simulink subsystem "rss_FaltEnFlgConfSens"  (R2023a)
settings: Solver=VariableStepAuto  StartTime=0.0  StopTime=10.0  RelTol=1e-3
undefined symbols (not defined in the file): Cdbl_numFaltDiaNum, ENM_SYS_STATUS, Gbol_flgFaltManEnFlg_C, Gu16_uComDiaDisblHiLvlConfTrs_C, Gu16_uComDiaDisblHiLvlRcvyTrs_C, Gu16_uComDiaDisblLoLvlConfTrs_C, Gu16_uComDiaDisblLoLvlRcvyTrs_C, Gu8_ctComDiaDisblHiLvlConfCnt_C, Gu8_ctComDiaDisblHiLvlRcvyCnt_C, Gu8_ctComDiaDisblLoLvlConfCnt_C, Gu8_ctComDiaDisblLoLvlRcvyCnt_C
libraries: simulink x3, lib_hysteresis_debounce x2
settings Model: Creator=xiaoqiang.yuan  LastModifiedBy=xiaoqiang.yuan

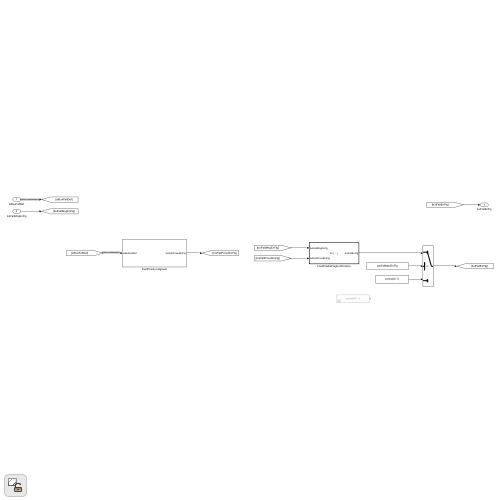
[thumbnail: Simulink's stored preview of the top-level diagram]
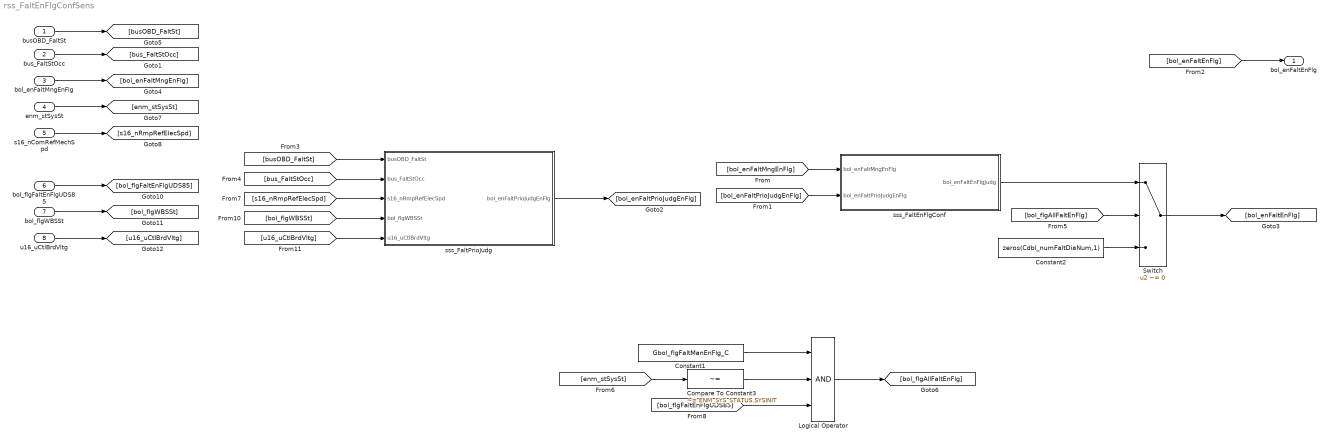
== system rss_FaltEnFlgConfSens ==
  busOBD_FaltSt : Inport
  bus_FaltStOcc : Inport  Port=2
  bol_enFaltMngEnFlg : Inport  Port=3
  enm_stSysSt : Inport  Port=4  OutDataTypeStr=Enum: ENM_SYS_STATUS
  s16_nComRefMechSpd : Inport  Port=5  OutDataTypeStr=dt_Standardize_s16p15b0
  bol_flgFaltEnFlgUDS85 : Inport  Port=6  OutDataTypeStr=boolean
  bol_flgWBSSt : Inport  Port=7  OutDataTypeStr=boolean
  u16_uCtlBrdVltg : Inport  Port=8  OutDataTypeStr=dt_Standardize_u16p15b0
  Compare To Constant3 : simulink/Logic and Bit Operations/Compare To Constant  relop=~=  const=ENM_SYS_STATUS.SYSINIT  OutDataTypeStr=boolean
  Constant1 : Constant  Value=Gbol_flgFaltManEnFlg_C
  Constant2 : Constant  Value=zeros(Cdbl_numFaltDiaNum,1)  OutDataTypeStr=boolean
  Logical Operator : Logic  Inputs=3  AllPortsSameDT=off  OutDataTypeStr=boolean
  Switch : Switch  Criteria=u2 ~= 0  SaturateOnIntegerOverflow=off  InputSameDT=off
  sss_FaltEnFlgConf : Subsystem  TreatAsAtomicUnit=on
      settings: RTWSystemCode=Nonreusable function
  sss_FaltPrioJudg : Subsystem
  bol_enFaltEnFlg : Outport
  wires:
  busOBD_FaltSt/1 -> [busOBD_FaltSt]
  [busOBD_FaltSt] -> sss_FaltPrioJudg/1(busOBD_FaltSt)
  sss_FaltPrioJudg/1(bol_enFaltPrioJudgEnFlg) -> [bol_enFaltPrioJudgEnFlg]
  [bol_enFaltMngEnFlg] -> sss_FaltEnFlgConf/1(bol_enFaltMngEnFlg)
  [bol_enFaltPrioJudgEnFlg] -> sss_FaltEnFlgConf/2(bol_enFaltPrioJudgEnFlg)
  [bol_enFaltEnFlg] -> bol_enFaltEnFlg/1
  bol_enFaltMngEnFlg/1 -> [bol_enFaltMngEnFlg]
  Constant2/1 -> Switch/3
  Switch/1 -> [bol_enFaltEnFlg]
  sss_FaltEnFlgConf/1(bol_enFaltEnFlgJudg) -> Switch/1
  bus_FaltStOcc/1 -> [bus_FaltStOcc]
  [bus_FaltStOcc] -> sss_FaltPrioJudg/2(bus_FaltStOcc)
  [bol_flgAllFaltEnFlg] -> Switch/2
  Constant1/1 -> Logical Operator/1
  enm_stSysSt/1 -> [enm_stSysSt]
  [enm_stSysSt] -> Compare To Constant3/1
  Compare To Constant3/1 -> Logical Operator/2
  Logical Operator/1 -> [bol_flgAllFaltEnFlg]
  s16_nComRefMechSpd/1 -> [s16_nRmpRefElecSpd]
  [s16_nRmpRefElecSpd] -> sss_FaltPrioJudg/3(s16_nRmpRefElecSpd)
  bol_flgFaltEnFlgUDS85/1 -> [bol_flgFaltEnFlgUDS85]
  bol_flgWBSSt/1 -> [bol_flgWBSSt]
  [bol_flgFaltEnFlgUDS85] -> Logical Operator/3
  u16_uCtlBrdVltg/1 -> [u16_uCtlBrdVltg]
  [bol_flgWBSSt] -> sss_FaltPrioJudg/4(bol_flgWBSSt)
  [u16_uCtlBrdVltg] -> sss_FaltPrioJudg/5(u16_uCtlBrdVltg)

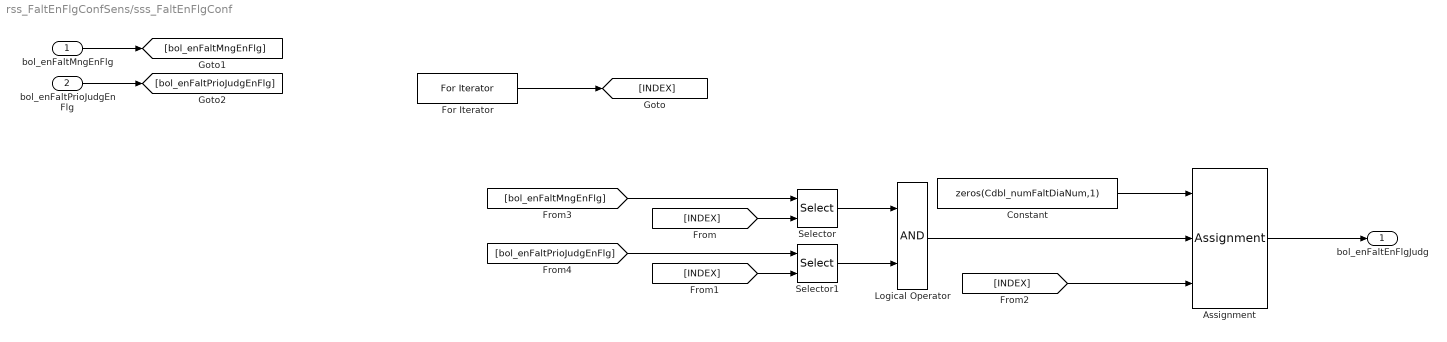
== system rss_FaltEnFlgConfSens/sss_FaltEnFlgConf ==
  bol_enFaltMngEnFlg : Inport
  bol_enFaltPrioJudgEnFlg : Inport  Port=2
  Assignment : Assignment  DiagnosticForDimensions=Warning  IndexOptions=Index vector (port)  Indices=1  OutputSizes=1
  Constant : Constant  Value=zeros(Cdbl_numFaltDiaNum,1)  OutDataTypeStr=boolean
  For Iterator : ForIterator  IterationLimit=Cdbl_numFaltDiaNum  IterationVariableDataType=uint8
  Logical Operator : Logic  AllPortsSameDT=off  OutDataTypeStr=boolean
  Selector : Selector  InputPortWidth=Cdbl_numFaltDiaNum  IndexOptions=Index vector (port)  Indices=[1 3]  OutputSizes=1
  Selector1 : Selector  InputPortWidth=Cdbl_numFaltDiaNum  IndexOptions=Index vector (port)  Indices=[1 3]  OutputSizes=1
  bol_enFaltEnFlgJudg : Outport
  wires:
  Assignment/1 -> bol_enFaltEnFlgJudg/1
  [bol_enFaltPrioJudgEnFlg] -> Selector1/1
  bol_enFaltPrioJudgEnFlg/1 -> [bol_enFaltPrioJudgEnFlg]
  bol_enFaltMngEnFlg/1 -> [bol_enFaltMngEnFlg]
  Selector/1 -> Logical Operator/1
  [bol_enFaltMngEnFlg] -> Selector/1
  For Iterator/1 -> [INDEX]
  [INDEX] -> Selector/2
  [INDEX] -> Selector1/2
  Selector1/1 -> Logical Operator/2
  Logical Operator/1 -> Assignment/2
  Constant/1 -> Assignment/1
  [INDEX] -> Assignment/3

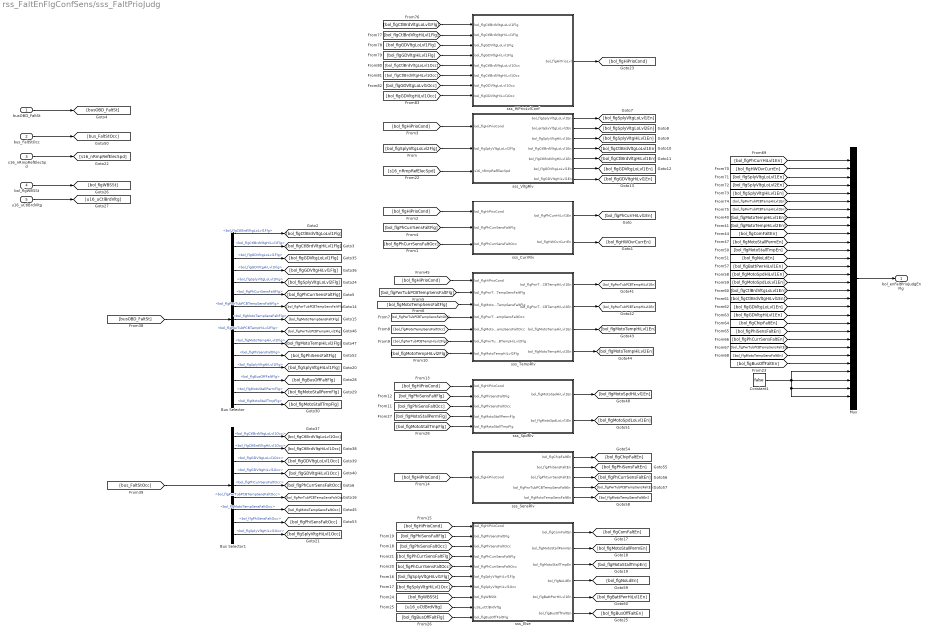
== system rss_FaltEnFlgConfSens/sss_FaltPrioJudg ==
  busOBD_FaltSt : Inport
  bus_FaltStOcc : Inport  Port=2
  s16_nRmpRefElecSpd : Inport  Port=3
  bol_flgWBSSt : Inport  Port=4
  u16_uCtlBrdVltg : Inport  Port=5
  Bus Selector : BusSelector  OutputSignals=bol_flgCtlBrdVltgLoLvl1Flg,bol_flgCtlBrdVltgHiLvl1Flg,bol_flgGDVltgLoLvl1Flg,bol_flgGDVltgHiLvl1Flg,bol_flgSplyVltgLoLvl2Flg,bol_flgPhCurrSensFaltFlg,bol_flgPwrTubPCBTempSensFaltFlg,bol_flgMotoTempSensFaltFlg,bol_flgPwrTubPCBTempHiLvl2Flg,bol_flgMotoTempHiLvl2Flg,bol_flgPhiSensFaltFlg,bol_flgSplyVltgHiLvl1Flg,bol_flgBusOffFaltFlg,bol_flgMotoStallPermFlg,bol_flgMotoStallTmpFlg
  Bus Selector1 : BusSelector  OutputSignals=bol_flgCtlBrdVltgLoLvl1Occ,bol_flgCtlBrdVltgHiLvl1Occ,bol_flgGDVltgLoLvl1Occ,bol_flgGDVltgHiLvl1Occ,bol_flgPhCurrSensFaltOcc,bol_flgPwrTubPCBTempSensFaltOcc,bol_flgMotoTempSensFaltOcc,bol_flgPhiSensFaltOcc,bol_flgSplyVltgHiLvl1Occ
  Constant1 : Constant  Value=false  OutDataTypeStr=boolean
  Mux : Mux  Inputs=30
  sss_CurrRlv : Subsystem
  sss_Else : Subsystem
  sss_HiPrioLvlConf : Subsystem
  sss_SensRlv : Subsystem
  sss_SpdRlv : Subsystem
  sss_TempRlv : Subsystem
  sss_VltgRlv : Subsystem
  bol_enFaltPrioJudgEnFlg : Outport
  wires:
  [bol_flgMotoStallTmpFlg] -> sss_SpdRlv/5(bol_flgMotoStallTmpFlg)
  [bol_flgMotoStallPermFlg] -> sss_SpdRlv/4(bol_flgMotoStallPermFlg)
  Bus Selector/15 -> [bol_flgMotoStallTmpFlg]  "<bol_flgMotoStallTmpFlg>"
  Bus Selector/14 -> [bol_flgMotoStallPermFlg]  "<bol_flgMotoStallPermFlg>"
  [bol_flgBusOffFaltEn] -> Mux/26
  sss_Else/6(bol_flgBusOffFaltEn) -> [bol_flgBusOffFaltEn]
  [bol_flgBusOffFaltFlg] -> sss_Else/10(bol_flgBusOffFaltFlg)
  Bus Selector/13 -> [bol_flgBusOffFaltFlg]  "<bol_flgBusOffFaltFlg>"
  [u16_uCtlBrdVltg] -> sss_Else/9(u16_uCtlBrdVltg)
  [bol_flgWBSSt] -> sss_Else/8(bol_flgWBSSt)
  u16_uCtlBrdVltg/1 -> [u16_uCtlBrdVltg]
  bol_flgWBSSt/1 -> [bol_flgWBSSt]
  [s16_nRmpRefElecSpd] -> sss_VltgRlv/3(s16_nRmpRefElecSpd)
  s16_nRmpRefElecSpd/1 -> [s16_nRmpRefElecSpd]
  [bol_flgSplyVltgHiLvl1Occ] -> sss_Else/7(bol_flgSplyVltgHiLvl1Occ)
  [bol_flgSplyVltgHiLvl1Flg] -> sss_Else/6(bol_flgSplyVltgHiLvl1Flg)
  [bol_flgPhCurrSensFaltOcc] -> sss_Else/5(bol_flgPhCurrSensFaltOcc)
  [bol_flgPhCurrSensFaltFlg] -> sss_Else/4(bol_flgPhCurrSensFaltFlg)
  [bol_flgPhiSensFaltOcc] -> sss_Else/3(bol_flgPhiSensFaltOcc)
  [bol_flgPhiSensFaltFlg] -> sss_Else/2(bol_flgPhiSensFaltFlg)
  Bus Selector1/9 -> [bol_flgSplyVltgHiLvl1Occ]  "<bol_flgSplyVltgHiLvl1Occ>"
  Bus Selector/12 -> [bol_flgSplyVltgHiLvl1Flg]  "<bol_flgSplyVltgHiLvl1Flg>"
  [bol_flgHiPrioCond] -> sss_Else/1(bol_flgHiPrioCond)
  sss_Else/5(bol_flgBattPwrHiLvl1En) -> [bol_flgBattPwrHiLvl1En]
  sss_Else/4(bol_flgNoLdEn) -> [bol_flgNoLdEn]
  sss_Else/3(bol_flgMotoStallTmpEn) -> [bol_flgMotoStallTmpEn]
  sss_Else/2(bol_flgMotoStallPermEn) -> [bol_flgMotoStallPermEn]
  sss_Else/1(bol_flgComFaltEn) -> [bol_flgComFaltEn]
  sss_SensRlv/5(bol_flgMotoTempSensFaltEn) -> [bol_flgMotoTempSensFaltEn]
  sss_SensRlv/4(bol_flgPwrTubPCBTempSensFaltEn) -> [bol_flgPwrTubPCBTempSensFaltEn]
  sss_SensRlv/3(bol_flgPhCurrSensFaltEn) -> [bol_flgPhCurrSensFaltEn]
  sss_SensRlv/2(bol_flgPhiSensFaltEn) -> [bol_flgPhiSensFaltEn]
  sss_SensRlv/1(bol_flgChipFaltEn) -> [bol_flgChipFaltEn]
  [bol_flgHiPrioCond] -> sss_SensRlv/1(bol_flgHiPrioCond)
  [bol_flgPhiSensFaltFlg] -> sss_SpdRlv/2(bol_flgPhiSensFaltFlg)
  [bol_flgPhiSensFaltOcc] -> sss_SpdRlv/3(bol_flgPhiSensFaltOcc)
  [bol_flgHiPrioCond] -> sss_SpdRlv/1(bol_flgHiPrioCond)
  Bus Selector1/8 -> [bol_flgPhiSensFaltOcc]  "<bol_flgPhiSensFaltOcc>"
  Bus Selector/11 -> [bol_flgPhiSensFaltFlg]  "<bol_flgPhiSensFaltFlg>"
  sss_SpdRlv/2(bol_flgMotoSpdLoLvl1En) -> [bol_flgMotoSpdLoLvl1En]
  sss_SpdRlv/1(bol_flgMotoSpdHiLvl1En) -> [bol_flgMotoSpdHiLvl1En]
  Bus Selector/10 -> [bol_flgMotoTempHiLvl2Flg]  "<bol_flgMotoTempHiLvl2Flg>"
  Bus Selector/9 -> [bol_flgPwrTubPCBTempHiLvl2Flg]  "<bol_flgPwrTubPCBTempHiLvl2Flg>"
  sss_TempRlv/1(bol_flgPwrTubPCBTempHiLvl1En) -> [bol_flgPwrTubPCBTempHiLvl1En]
  sss_TempRlv/2(bol_flgPwrTubPCBTempHiLvl2En) -> [bol_flgPwrTubPCBTempHiLvl2En]
  sss_TempRlv/3(bol_flgMotoTempHiLvl1En) -> [bol_flgMotoTempHiLvl1En]
  sss_TempRlv/4(bol_flgMotoTempHiLvl2En) -> [bol_flgMotoTempHiLvl2En]
  [bol_flgMotoTempHiLvl2Flg] -> sss_TempRlv/7(bol_flgMotoTempHiLvl2Flg)
  [bol_flgPwrTubPCBTempHiLvl2Flg] -> sss_TempRlv/6(bol_flgPwrTubPCBTempHiLvl2Flg)
  [bol_flgMotoTempSensFaltOcc] -> sss_TempRlv/5(bol_flgMotoTempSensFaltOcc)
  [bol_flgPwrTubPCBTempSensFaltOcc] -> sss_TempRlv/4(bol_flgPwrTubPCBTempSensFaltOcc)
  [bol_flgMotoTempSensFaltFlg] -> sss_TempRlv/3(bol_flgMotoTempSensFaltFlg)
  [bol_flgPwrTubPCBTempSensFaltFlg] -> sss_TempRlv/2(bol_flgPwrTubPCBTempSensFaltFlg)
  Bus Selector1/7 -> [bol_flgMotoTempSensFaltOcc]  "<bol_flgMotoTempSensFaltOcc>"
  Bus Selector1/6 -> [bol_flgPwrTubPCBTempSensFaltOcc]  "<bol_flgPwrTubPCBTempSensFaltOcc>"
  Bus Selector/8 -> [bol_flgMotoTempSensFaltFlg]  "<bol_flgMotoTempSensFaltFlg>"
  Bus Selector/7 -> [bol_flgPwrTubPCBTempSensFaltFlg]  "<bol_flgPwrTubPCBTempSensFaltFlg>"
  [bol_flgHiPrioCond] -> sss_CurrRlv/1(bol_flgHiPrioCond)
  [bol_flgPhCurrSensFaltOcc] -> sss_CurrRlv/3(bol_flgPhCurrSensFaltOcc)
  [bol_flgPhCurrSensFaltFlg] -> sss_CurrRlv/2(bol_flgPhCurrSensFaltFlg)
  Bus Selector1/5 -> [bol_flgPhCurrSensFaltOcc]  "<bol_flgPhCurrSensFaltOcc>"
  Bus Selector/6 -> [bol_flgPhCurrSensFaltFlg]  "<bol_flgPhCurrSensFaltFlg>"
  [bol_flgSplyVltgLoLvl2Flg] -> sss_VltgRlv/2(bol_flgSplyVltgLoLvl2Flg)
  Bus Selector/5 -> [bol_flgSplyVltgLoLvl2Flg]  "<bol_flgSplyVltgLoLvl2Flg>"
  [bol_flgHiPrioCond] -> sss_VltgRlv/1(bol_flgHiPrioCond)
  sss_VltgRlv/7(bol_flgGDVltgHiLvl1En) -> [bol_flgGDVltgHiLvl1En]
  sss_VltgRlv/6(bol_flgGDVltgLoLvl1En) -> [bol_flgGDVltgLoLvl1En]
  sss_VltgRlv/5(bol_flgCtlBrdVltgHiLvl1En) -> [bol_flgCtlBrdVltgHiLvl1En]
  sss_VltgRlv/4(bol_flgCtlBrdVltgLoLvl1En) -> [bol_flgCtlBrdVltgLoLvl1En]
  sss_VltgRlv/3(bol_flgSplyVltgHiLvl1En) -> [bol_flgSplyVltgHiLvl1En]
  sss_VltgRlv/2(bol_enSplyVltgLoLvl2En) -> [bol_flgSplyVltgLoLvl2En]
  sss_VltgRlv/1(bol_flgSplyVltgLoLvl1En) -> [bol_flgSplyVltgLoLvl1En]
  Mux/1 -> bol_enFaltPrioJudgEnFlg/1
  [bol_flgGDVltgHiLvl1Occ] -> sss_HiPrioLvlConf/8(bol_flgGDVltgHiLvl1Occ)
  [bol_flgGDVltgLoLvl1Occ] -> sss_HiPrioLvlConf/7(bol_flgGDVltgLoLvl1Occ)
  [bol_flgCtlBrdVltgHiLvl1Occ] -> sss_HiPrioLvlConf/6(bol_flgCtlBrdVltgHiLvl1Occ)
  [bol_flgCtlBrdVltgLoLvl1Occ] -> sss_HiPrioLvlConf/5(bol_flgCtlBrdVltgLoLvl1Occ)
  [bol_flgGDVltgHiLvl1Flg] -> sss_HiPrioLvlConf/4(bol_flgGDVltgHiLvl1Flg)
  [bol_flgGDVltgLoLvl1Flg] -> sss_HiPrioLvlConf/3(bol_flgGDVltgLoLvl1Flg)
  [bol_flgCtlBrdVltgHiLvl1Flg] -> sss_HiPrioLvlConf/2(bol_flgCtlBrdVltgHiLvl1Flg)
  [bol_flgCtlBrdVltgLoLvl1Flg] -> sss_HiPrioLvlConf/1(bol_flgCtlBrdVltgLoLvl1Flg)
  Bus Selector1/4 -> [bol_flgGDVltgHiLvl1Occ]  "<bol_flgGDVltgHiLvl1Occ>"
  Bus Selector1/3 -> [bol_flgGDVltgLoLvl1Occ]  "<bol_flgGDVltgLoLvl1Occ>"
  Bus Selector1/2 -> [bol_flgCtlBrdVltgHiLvl1Occ]  "<bol_flgCtlBrdVltgHiLvl1Occ>"
  Bus Selector1/1 -> [bol_flgCtlBrdVltgLoLvl1Occ]  "<bol_flgCtlBrdVltgLoLvl1Occ>"
  [bol_flgGDVltgHiLvl1En] -> Mux/20
  [bol_flgMotoStallPermEn] -> Mux/11
  [bol_flgPhCurrSensFaltEn] -> Mux/23
  [bol_flgCtlBrdVltgHiLvl1En] -> Mux/18
  [bol_flgMotoStallTmpEn] -> Mux/12
  [bol_flgMotoSpdLoLvl1En] -> Mux/16
  [bol_flgCtlBrdVltgLoLvl1En] -> Mux/17
  [bol_flgBattPwrHiLvl1En] -> Mux/14
  [bol_flgNoLdEn] -> Mux/13
  [bol_flgPhCurrHiLvl1En] -> Mux/1
  [bol_flgPhiSensFaltEn] -> Mux/22
  [bol_flgMotoTempHiLvl1En] -> Mux/8
  [bol_flgMotoTempHiLvl2En] -> Mux/9
  [bol_flgChipFaltEn] -> Mux/21
  [bol_flgHWOvrCurrEn] -> Mux/2
  [bol_flgPwrTubPCBTempHiLvl1En] -> Mux/6
  [bol_flgComFaltEn] -> Mux/10
  [bol_flgPwrTubPCBTempHiLvl2En] -> Mux/7
  [bol_flgMotoSpdHiLvl1En] -> Mux/15
  [bol_flgSplyVltgHiLvl1En] -> Mux/5
  [bol_flgPwrTubPCBTempSensFaltEn] -> Mux/24
  [bol_flgGDVltgLoLvl1En] -> Mux/19
  [bol_flgSplyVltgLoLvl2En] -> Mux/4
  [bol_flgMotoTempSensFaltEn] -> Mux/25
  [bol_flgSplyVltgLoLvl1En] -> Mux/3
  Constant1/1 -> Mux/30, Mux/29, Mux/28, Mux/27
  [bus_FaltStOcc] -> Bus Selector1/1
  bus_FaltStOcc/1 -> [bus_FaltStOcc]
  sss_HiPrioLvlConf/1(bol_flgHiPrioLvl) -> [bol_flgHiPrioCond]
  [bol_flgHiPrioCond] -> sss_TempRlv/1(bol_flgHiPrioCond)
  sss_CurrRlv/2(bol_flgHWOvrCurrEn) -> [bol_flgHWOvrCurrEn]
  sss_CurrRlv/1(bol_flgPhCurrHiLvl1En) -> [bol_flgPhCurrHiLvl1En]
  Bus Selector/4 -> [bol_flgGDVltgHiLvl1Flg]  "<bol_flgGDVltgHiLvl1Flg>"
  Bus Selector/3 -> [bol_flgGDVltgLoLvl1Flg]  "<bol_flgGDVltgLoLvl1Flg>"
  busOBD_FaltSt/1 -> [busOBD_FaltSt]
  Bus Selector/2 -> [bol_flgCtlBrdVltgHiLvl1Flg]  "<bol_flgCtlBrdVltgHiLvl1Flg>"
  Bus Selector/1 -> [bol_flgCtlBrdVltgLoLvl1Flg]  "<bol_flgCtlBrdVltgLoLvl1Flg>"
  [busOBD_FaltSt] -> Bus Selector/1

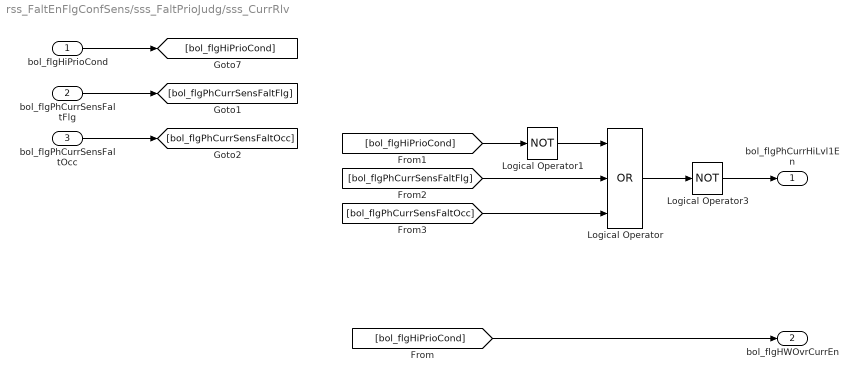
== system rss_FaltEnFlgConfSens/sss_FaltPrioJudg/sss_CurrRlv ==
  bol_flgHiPrioCond : Inport
  bol_flgPhCurrSensFaltFlg : Inport  Port=2
  bol_flgPhCurrSensFaltOcc : Inport  Port=3
  Logical Operator : Logic  Operator=OR  Inputs=3  AllPortsSameDT=off  OutDataTypeStr=boolean
  Logical Operator1 : Logic  Operator=NOT  AllPortsSameDT=off  OutDataTypeStr=boolean
  Logical Operator3 : Logic  Operator=NOT  AllPortsSameDT=off  OutDataTypeStr=boolean
  bol_flgPhCurrHiLvl1En : Outport
  bol_flgHWOvrCurrEn : Outport  Port=2
  wires:
  [bol_flgPhCurrSensFaltOcc] -> Logical Operator/3
  [bol_flgHiPrioCond] -> Logical Operator1/1
  Logical Operator3/1 -> bol_flgPhCurrHiLvl1En/1
  bol_flgPhCurrSensFaltOcc/1 -> [bol_flgPhCurrSensFaltOcc]
  bol_flgPhCurrSensFaltFlg/1 -> [bol_flgPhCurrSensFaltFlg]
  bol_flgHiPrioCond/1 -> [bol_flgHiPrioCond]
  Logical Operator/1 -> Logical Operator3/1
  [bol_flgHiPrioCond] -> bol_flgHWOvrCurrEn/1
  [bol_flgPhCurrSensFaltFlg] -> Logical Operator/2
  Logical Operator1/1 -> Logical Operator/1

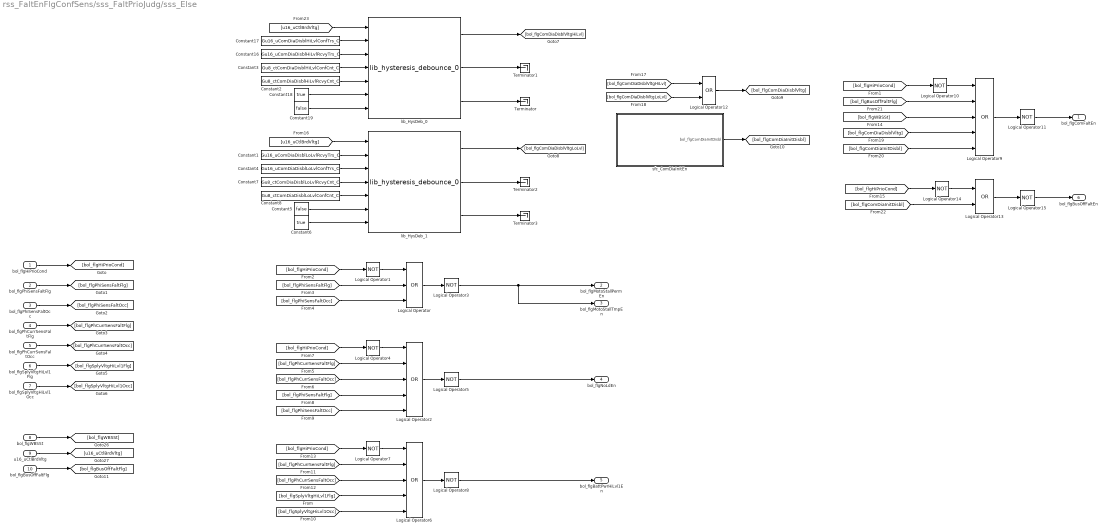
== system rss_FaltEnFlgConfSens/sss_FaltPrioJudg/sss_Else ==
  bol_flgHiPrioCond : Inport
  bol_flgPhiSensFaltFlg : Inport  Port=2
  bol_flgPhiSensFaltOcc : Inport  Port=3
  bol_flgPhCurrSensFaltFlg : Inport  Port=4
  bol_flgPhCurrSensFaltOcc : Inport  Port=5
  bol_flgSplyVltgHiLvl1Flg : Inport  Port=6
  bol_flgSplyVltgHiLvl1Occ : Inport  Port=7
  bol_flgWBSSt : Inport  Port=8
  u16_uCtlBrdVltg : Inport  Port=9
  bol_flgBusOffFaltFlg : Inport  Port=10
  Constant1 : Constant  Value=Gu16_uComDiaDisblLoLvlRcvyTrs_C
  Constant16 : Constant  Value=Gu16_uComDiaDisblHiLvlRcvyTrs_C
  Constant17 : Constant  Value=Gu16_uComDiaDisblHiLvlConfTrs_C
  Constant18 : Constant  Value=true  OutDataTypeStr=boolean
  Constant19 : Constant  Value=false  OutDataTypeStr=boolean
  Constant2 : Constant  Value=Gu8_ctComDiaDisblHiLvlRcvyCnt_C
  Constant3 : Constant  Value=Gu8_ctComDiaDisblHiLvlConfCnt_C
  Constant4 : Constant  Value=Gu16_uComDiaDisblLoLvlConfTrs_C
  Constant5 : Constant  Value=false  OutDataTypeStr=boolean
  Constant6 : Constant  Value=true  OutDataTypeStr=boolean
  Constant7 : Constant  Value=Gu8_ctComDiaDisblLoLvlRcvyCnt_C
  Constant8 : Constant  Value=Gu8_ctComDiaDisblLoLvlConfCnt_C
  Logical Operator : Logic  Operator=OR  Inputs=3  AllPortsSameDT=off  OutDataTypeStr=boolean
  Logical Operator{1,3..5,7..8,10..11,14..15} (10 alike) : Logic  Operator=NOT  AllPortsSameDT=off  OutDataTypeStr=boolean
  Logical Operator12 : Logic  Operator=OR  AllPortsSameDT=off  OutDataTypeStr=boolean
  Logical Operator13 : Logic  Operator=OR  AllPortsSameDT=off  OutDataTypeStr=boolean
  Logical Operator2 : Logic  Operator=OR  Inputs=5  AllPortsSameDT=off  OutDataTypeStr=boolean
  Logical Operator6 : Logic  Operator=OR  Inputs=5  AllPortsSameDT=off  OutDataTypeStr=boolean
  Logical Operator9 : Logic  Operator=OR  Inputs=5  AllPortsSameDT=off  OutDataTypeStr=boolean
  Terminator{,1..3} (4 alike) : Terminator
  lib_HysDeb_0 : lib_hysteresis_debounce/lib_hysteresis_debounce_0  lb_parInitOutp=0
  lib_HysDeb_1 : lib_hysteresis_debounce/lib_hysteresis_debounce_0  lb_parInitOutp=0
  sfc_ComDiaInitEn : Stateflow chart  TreatAsAtomicUnit=on
  bol_flgComFaltEn : Outport
  bol_flgMotoStallPermEn : Outport  Port=2
  bol_flgMotoStallTmpEn : Outport  Port=3
  bol_flgNoLdEn : Outport  Port=4
  bol_flgBattPwrHiLvl1En : Outport  Port=5
  bol_flgBusOffFaltEn : Outport  Port=6
  wires:
  Logical Operator15/1 -> bol_flgBusOffFaltEn/1
  Logical Operator14/1 -> Logical Operator13/1
  [bol_flgHiPrioCond] -> Logical Operator14/1
  Logical Operator13/1 -> Logical Operator15/1
  [bol_flgComDiaInitDisbl] -> Logical Operator13/2
  [bol_flgBusOffFaltFlg] -> Logical Operator9/2
  bol_flgBusOffFaltFlg/1 -> [bol_flgBusOffFaltFlg]
  sfc_ComDiaInitEn/1(bol_flgComDiaInitDisbl) -> [bol_flgComDiaInitDisbl]
  [bol_flgComDiaInitDisbl] -> Logical Operator9/5
  Logical Operator11/1 -> bol_flgComFaltEn/1
  [bol_flgComDiaDisblVltg] -> Logical Operator9/4
  Logical Operator12/1 -> [bol_flgComDiaDisblVltg]
  [bol_flgComDiaDisblVltgHiLvl] -> Logical Operator12/1
  [bol_flgComDiaDisblVltgLoLvl] -> Logical Operator12/2
  lib_HysDeb_1/2 -> Terminator2/1
  Constant6/1 -> lib_HysDeb_1/7
  lib_HysDeb_1/1 -> [bol_flgComDiaDisblVltgLoLvl]
  Constant7/1 -> lib_HysDeb_1/4
  Constant1/1 -> lib_HysDeb_1/2
  Constant5/1 -> lib_HysDeb_1/6
  Constant4/1 -> lib_HysDeb_1/3
  [u16_uCtlBrdVltg] -> lib_HysDeb_1/1
  Constant8/1 -> lib_HysDeb_1/5
  lib_HysDeb_1/3 -> Terminator3/1
  [u16_uCtlBrdVltg] -> lib_HysDeb_0/1
  lib_HysDeb_0/1 -> [bol_flgComDiaDisblVltgHiLvl]
  Constant19/1 -> lib_HysDeb_0/7
  Constant18/1 -> lib_HysDeb_0/6
  Constant16/1 -> lib_HysDeb_0/3
  lib_HysDeb_0/2 -> Terminator1/1
  lib_HysDeb_0/3 -> Terminator/1
  Constant3/1 -> lib_HysDeb_0/4
  Constant2/1 -> lib_HysDeb_0/5
  Constant17/1 -> lib_HysDeb_0/2
  Logical Operator10/1 -> Logical Operator9/1
  [bol_flgHiPrioCond] -> Logical Operator10/1
  Logical Operator9/1 -> Logical Operator11/1
  [bol_flgWBSSt] -> Logical Operator9/3
  bol_flgWBSSt/1 -> [bol_flgWBSSt]
  u16_uCtlBrdVltg/1 -> [u16_uCtlBrdVltg]
  [bol_flgSplyVltgHiLvl1Flg] -> Logical Operator6/4
  Logical Operator8/1 -> bol_flgBattPwrHiLvl1En/1
  [bol_flgHiPrioCond] -> Logical Operator7/1
  Logical Operator6/1 -> Logical Operator8/1
  [bol_flgPhCurrSensFaltFlg] -> Logical Operator6/2
  [bol_flgPhCurrSensFaltOcc] -> Logical Operator6/3
  Logical Operator7/1 -> Logical Operator6/1
  [bol_flgSplyVltgHiLvl1Occ] -> Logical Operator6/5
  bol_flgSplyVltgHiLvl1Occ/1 -> [bol_flgSplyVltgHiLvl1Occ]
  bol_flgSplyVltgHiLvl1Flg/1 -> [bol_flgSplyVltgHiLvl1Flg]
  [bol_flgPhiSensFaltOcc] -> Logical Operator2/5
  [bol_flgPhiSensFaltFlg] -> Logical Operator2/4
  [bol_flgHiPrioCond] -> Logical Operator4/1
  Logical Operator2/1 -> Logical Operator5/1
  Logical Operator5/1 -> bol_flgNoLdEn/1
  [bol_flgPhCurrSensFaltOcc] -> Logical Operator2/3
  [bol_flgPhCurrSensFaltFlg] -> Logical Operator2/2
  Logical Operator4/1 -> Logical Operator2/1
  bol_flgPhCurrSensFaltOcc/1 -> [bol_flgPhCurrSensFaltOcc]
  bol_flgPhCurrSensFaltFlg/1 -> [bol_flgPhCurrSensFaltFlg]
  Logical Operator3/1 -> bol_flgMotoStallPermEn/1, bol_flgMotoStallTmpEn/1
  [bol_flgPhiSensFaltOcc] -> Logical Operator/3
  [bol_flgPhiSensFaltFlg] -> Logical Operator/2
  bol_flgPhiSensFaltOcc/1 -> [bol_flgPhiSensFaltOcc]
  bol_flgPhiSensFaltFlg/1 -> [bol_flgPhiSensFaltFlg]
  Logical Operator/1 -> Logical Operator3/1
  [bol_flgHiPrioCond] -> Logical Operator1/1
  Logical Operator1/1 -> Logical Operator/1
  bol_flgHiPrioCond/1 -> [bol_flgHiPrioCond]

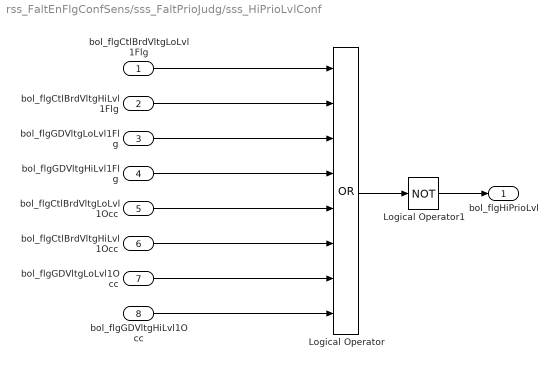
== system rss_FaltEnFlgConfSens/sss_FaltPrioJudg/sss_HiPrioLvlConf ==
  bol_flgCtlBrdVltgLoLvl1Flg : Inport
  bol_flgCtlBrdVltgHiLvl1Flg : Inport  Port=2
  bol_flgGDVltgLoLvl1Flg : Inport  Port=3
  bol_flgGDVltgHiLvl1Flg : Inport  Port=4
  bol_flgCtlBrdVltgLoLvl1Occ : Inport  Port=5
  bol_flgCtlBrdVltgHiLvl1Occ : Inport  Port=6
  bol_flgGDVltgLoLvl1Occ : Inport  Port=7
  bol_flgGDVltgHiLvl1Occ : Inport  Port=8
  Logical Operator : Logic  Operator=OR  Inputs=8  AllPortsSameDT=off  OutDataTypeStr=boolean
  Logical Operator1 : Logic  Operator=NOT  AllPortsSameDT=off  OutDataTypeStr=boolean
  bol_flgHiPrioLvl : Outport
  wires:
  Logical Operator1/1 -> bol_flgHiPrioLvl/1
  Logical Operator/1 -> Logical Operator1/1
  bol_flgGDVltgHiLvl1Occ/1 -> Logical Operator/8
  bol_flgGDVltgLoLvl1Occ/1 -> Logical Operator/7
  bol_flgCtlBrdVltgHiLvl1Occ/1 -> Logical Operator/6
  bol_flgCtlBrdVltgLoLvl1Occ/1 -> Logical Operator/5
  bol_flgGDVltgHiLvl1Flg/1 -> Logical Operator/4
  bol_flgGDVltgLoLvl1Flg/1 -> Logical Operator/3
  bol_flgCtlBrdVltgHiLvl1Flg/1 -> Logical Operator/2
  bol_flgCtlBrdVltgLoLvl1Flg/1 -> Logical Operator/1

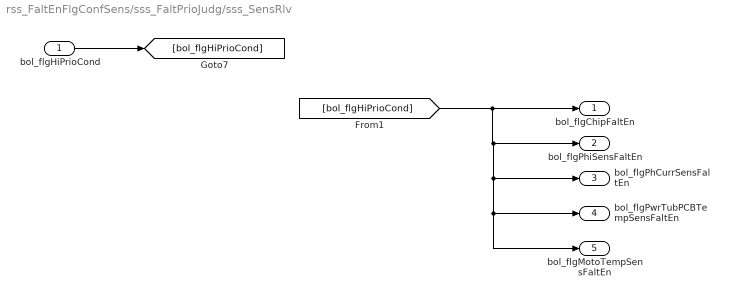
== system rss_FaltEnFlgConfSens/sss_FaltPrioJudg/sss_SensRlv ==
  bol_flgHiPrioCond : Inport
  bol_flgChipFaltEn : Outport
  bol_flgPhiSensFaltEn : Outport  Port=2
  bol_flgPhCurrSensFaltEn : Outport  Port=3
  bol_flgPwrTubPCBTempSensFaltEn : Outport  Port=4
  bol_flgMotoTempSensFaltEn : Outport  Port=5
  wires:
  [bol_flgHiPrioCond] -> bol_flgChipFaltEn/1, bol_flgPhiSensFaltEn/1, bol_flgPhCurrSensFaltEn/1, bol_flgMotoTempSensFaltEn/1, bol_flgPwrTubPCBTempSensFaltEn/1
  bol_flgHiPrioCond/1 -> [bol_flgHiPrioCond]

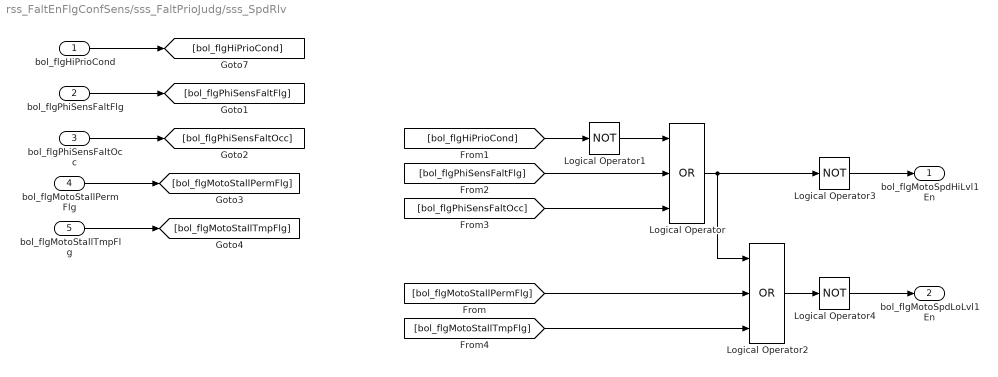
== system rss_FaltEnFlgConfSens/sss_FaltPrioJudg/sss_SpdRlv ==
  bol_flgHiPrioCond : Inport
  bol_flgPhiSensFaltFlg : Inport  Port=2
  bol_flgPhiSensFaltOcc : Inport  Port=3
  bol_flgMotoStallPermFlg : Inport  Port=4
  bol_flgMotoStallTmpFlg : Inport  Port=5
  Logical Operator : Logic  Operator=OR  Inputs=3  AllPortsSameDT=off  OutDataTypeStr=boolean
  Logical Operator1 : Logic  Operator=NOT  AllPortsSameDT=off  OutDataTypeStr=boolean
  Logical Operator2 : Logic  Operator=OR  Inputs=3  AllPortsSameDT=off  OutDataTypeStr=boolean
  Logical Operator3 : Logic  Operator=NOT  AllPortsSameDT=off  OutDataTypeStr=boolean
  Logical Operator4 : Logic  Operator=NOT  AllPortsSameDT=off  OutDataTypeStr=boolean
  bol_flgMotoSpdHiLvl1En : Outport
  bol_flgMotoSpdLoLvl1En : Outport  Port=2
  wires:
  Logical Operator4/1 -> bol_flgMotoSpdLoLvl1En/1
  Logical Operator2/1 -> Logical Operator4/1
  [bol_flgMotoStallTmpFlg] -> Logical Operator2/3
  [bol_flgMotoStallPermFlg] -> Logical Operator2/2
  bol_flgMotoStallTmpFlg/1 -> [bol_flgMotoStallTmpFlg]
  bol_flgMotoStallPermFlg/1 -> [bol_flgMotoStallPermFlg]
  Logical Operator1/1 -> Logical Operator/1
  [bol_flgPhiSensFaltFlg] -> Logical Operator/2
  Logical Operator/1 -> Logical Operator3/1, Logical Operator2/1
  bol_flgHiPrioCond/1 -> [bol_flgHiPrioCond]
  bol_flgPhiSensFaltFlg/1 -> [bol_flgPhiSensFaltFlg]
  bol_flgPhiSensFaltOcc/1 -> [bol_flgPhiSensFaltOcc]
  Logical Operator3/1 -> bol_flgMotoSpdHiLvl1En/1
  [bol_flgHiPrioCond] -> Logical Operator1/1
  [bol_flgPhiSensFaltOcc] -> Logical Operator/3

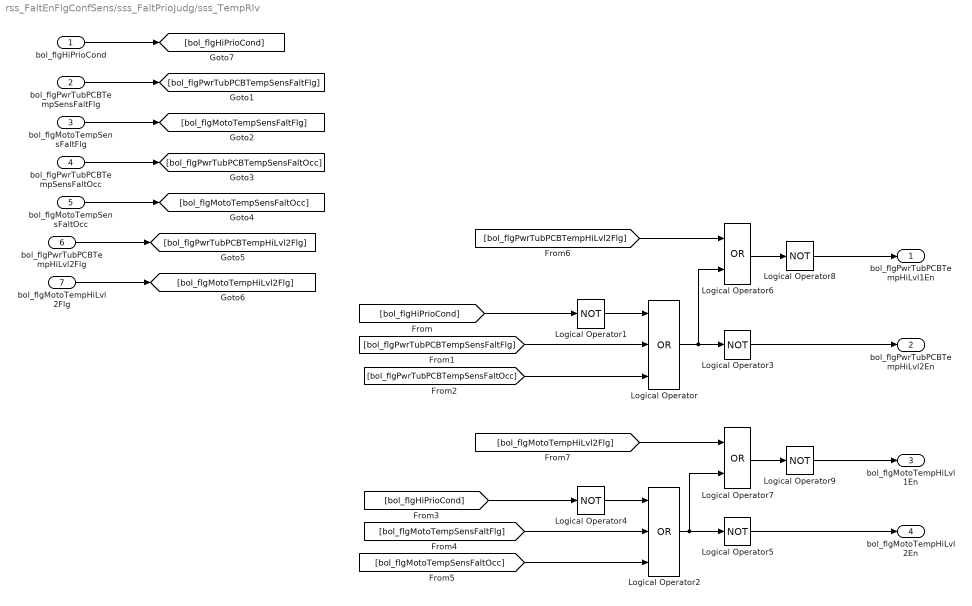
== system rss_FaltEnFlgConfSens/sss_FaltPrioJudg/sss_TempRlv ==
  bol_flgHiPrioCond : Inport
  bol_flgPwrTubPCBTempSensFaltFlg : Inport  Port=2
  bol_flgMotoTempSensFaltFlg : Inport  Port=3
  bol_flgPwrTubPCBTempSensFaltOcc : Inport  Port=4
  bol_flgMotoTempSensFaltOcc : Inport  Port=5
  bol_flgPwrTubPCBTempHiLvl2Flg : Inport  Port=6
  bol_flgMotoTempHiLvl2Flg : Inport  Port=7
  Logical Operator : Logic  Operator=OR  Inputs=3  AllPortsSameDT=off  OutDataTypeStr=boolean
  Logical Operator{1,3..5,8..9} (6 alike) : Logic  Operator=NOT  AllPortsSameDT=off  OutDataTypeStr=boolean
  Logical Operator2 : Logic  Operator=OR  Inputs=3  AllPortsSameDT=off  OutDataTypeStr=boolean
  Logical Operator6 : Logic  Operator=OR  AllPortsSameDT=off  OutDataTypeStr=boolean
  Logical Operator7 : Logic  Operator=OR  AllPortsSameDT=off  OutDataTypeStr=boolean
  bol_flgPwrTubPCBTempHiLvl1En : Outport
  bol_flgPwrTubPCBTempHiLvl2En : Outport  Port=2
  bol_flgMotoTempHiLvl1En : Outport  Port=3
  bol_flgMotoTempHiLvl2En : Outport  Port=4
  wires:
  Logical Operator9/1 -> bol_flgMotoTempHiLvl1En/1
  Logical Operator8/1 -> bol_flgPwrTubPCBTempHiLvl1En/1
  Logical Operator7/1 -> Logical Operator9/1
  [bol_flgMotoTempHiLvl2Flg] -> Logical Operator7/1
  Logical Operator6/1 -> Logical Operator8/1
  [bol_flgPwrTubPCBTempHiLvl2Flg] -> Logical Operator6/1
  bol_flgMotoTempHiLvl2Flg/1 -> [bol_flgMotoTempHiLvl2Flg]
  bol_flgPwrTubPCBTempHiLvl2Flg/1 -> [bol_flgPwrTubPCBTempHiLvl2Flg]
  Logical Operator2/1 -> Logical Operator5/1, Logical Operator7/2
  [bol_flgHiPrioCond] -> Logical Operator4/1
  [bol_flgMotoTempSensFaltFlg] -> Logical Operator2/2
  Logical Operator4/1 -> Logical Operator2/1
  Logical Operator5/1 -> bol_flgMotoTempHiLvl2En/1
  [bol_flgMotoTempSensFaltOcc] -> Logical Operator2/3
  Logical Operator3/1 -> bol_flgPwrTubPCBTempHiLvl2En/1
  [bol_flgHiPrioCond] -> Logical Operator1/1
  bol_flgMotoTempSensFaltOcc/1 -> [bol_flgMotoTempSensFaltOcc]
  bol_flgPwrTubPCBTempSensFaltOcc/1 -> [bol_flgPwrTubPCBTempSensFaltOcc]
  bol_flgMotoTempSensFaltFlg/1 -> [bol_flgMotoTempSensFaltFlg]
  bol_flgPwrTubPCBTempSensFaltFlg/1 -> [bol_flgPwrTubPCBTempSensFaltFlg]
  bol_flgHiPrioCond/1 -> [bol_flgHiPrioCond]
  [bol_flgPwrTubPCBTempSensFaltOcc] -> Logical Operator/3
  Logical Operator1/1 -> Logical Operator/1
  Logical Operator/1 -> Logical Operator3/1, Logical Operator6/2
  [bol_flgPwrTubPCBTempSensFaltFlg] -> Logical Operator/2

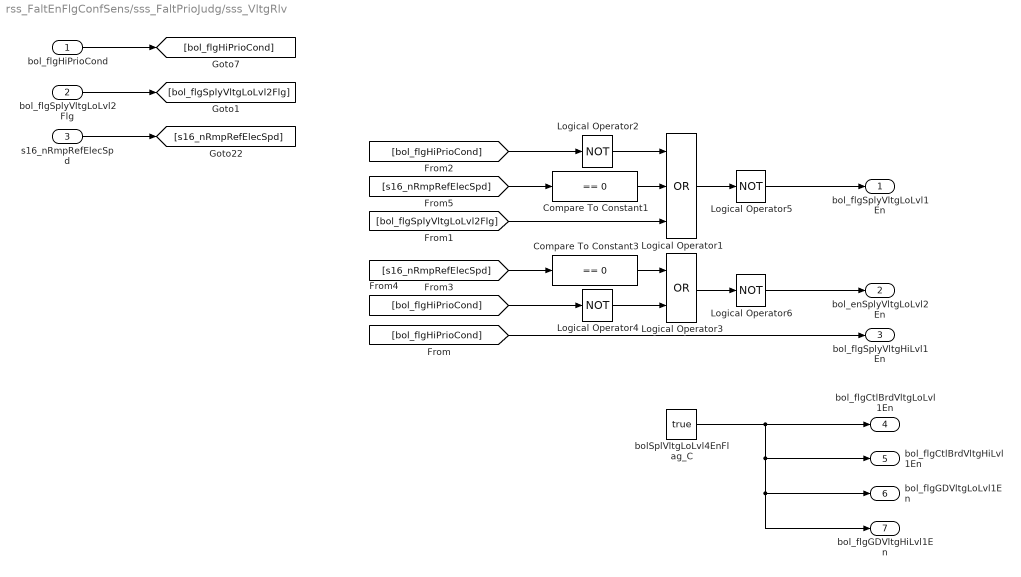
== system rss_FaltEnFlgConfSens/sss_FaltPrioJudg/sss_VltgRlv ==
  bol_flgHiPrioCond : Inport
  bol_flgSplyVltgLoLvl2Flg : Inport  Port=2
  s16_nRmpRefElecSpd : Inport  Port=3
  Compare To Constant1 : simulink/Logic and Bit Operations/Compare To Constant  relop===  const=0  OutDataTypeStr=boolean
  Compare To Constant3 : simulink/Logic and Bit Operations/Compare To Constant  relop===  const=0  OutDataTypeStr=boolean
  Logical Operator1 : Logic  Operator=OR  Inputs=3  AllPortsSameDT=off  OutDataTypeStr=boolean
  Logical Operator{2,4..6} (4 alike) : Logic  Operator=NOT  AllPortsSameDT=off  OutDataTypeStr=boolean
  Logical Operator3 : Logic  Operator=OR  AllPortsSameDT=off  OutDataTypeStr=boolean
  bolSplVltgLoLvl4EnFlag_C : Constant  Value=true
  bol_flgSplyVltgLoLvl1En : Outport
  bol_enSplyVltgLoLvl2En : Outport  Port=2
  bol_flgSplyVltgHiLvl1En : Outport  Port=3
  bol_flgCtlBrdVltgLoLvl1En : Outport  Port=4
  bol_flgCtlBrdVltgHiLvl1En : Outport  Port=5
  bol_flgGDVltgLoLvl1En : Outport  Port=6
  bol_flgGDVltgHiLvl1En : Outport  Port=7
  wires:
  Compare To Constant1/1 -> Logical Operator1/2
  [s16_nRmpRefElecSpd] -> Compare To Constant1/1
  [bol_flgSplyVltgLoLvl2Flg] -> Logical Operator1/3
  Logical Operator6/1 -> bol_enSplyVltgLoLvl2En/1
  Logical Operator4/1 -> Logical Operator3/2
  [bol_flgHiPrioCond] -> Logical Operator4/1
  Compare To Constant3/1 -> Logical Operator3/1
  Logical Operator3/1 -> Logical Operator6/1
  [s16_nRmpRefElecSpd] -> Compare To Constant3/1
  s16_nRmpRefElecSpd/1 -> [s16_nRmpRefElecSpd]
  Logical Operator5/1 -> bol_flgSplyVltgLoLvl1En/1
  Logical Operator1/1 -> Logical Operator5/1
  Logical Operator2/1 -> Logical Operator1/1
  [bol_flgHiPrioCond] -> Logical Operator2/1
  bol_flgSplyVltgLoLvl2Flg/1 -> [bol_flgSplyVltgLoLvl2Flg]
  [bol_flgHiPrioCond] -> bol_flgSplyVltgHiLvl1En/1
  bol_flgHiPrioCond/1 -> [bol_flgHiPrioCond]
  bolSplVltgLoLvl4EnFlag_C/1 -> bol_flgCtlBrdVltgLoLvl1En/1, bol_flgGDVltgHiLvl1En/1, bol_flgGDVltgLoLvl1En/1, bol_flgCtlBrdVltgHiLvl1En/1

== stateflow chart rss_FaltEnFlgConfSens/sss_FaltPrioJudg/sss_Else/sfc_ComDiaInitEn ==
  state INITDISBL
    en:
    bol_flgComDiaInitDisbl = true;
    u16_ctInitDisblCnt = 0;
    du:
    u16_ctInitDisblCnt = u16_ctInitDisblCnt + 1;
    ex:
    u16_ctInitDisblCnt = 0;
  state INITEN
    du:
    bol_flgComDiaInitDisbl = false;
  (default) -> INITDISBL
  INITDISBL -> INITEN : [u16_ctInitDisblCnt>= Gu16_ctInitDisblCnt_C]
  data: u16_ctInitDisblCnt local uint16; bol_flgComDiaInitDisbl output boolean; Gu16_ctInitDisblCnt_C parameter
